simulink model "Problem3"  (R2020b)
settings: Solver=VariableStepAuto  StartTime=0.0  StopTime=0.1  RelTol=1e-3
settings Model: Creator=Saqlain  LastModifiedBy=Acer

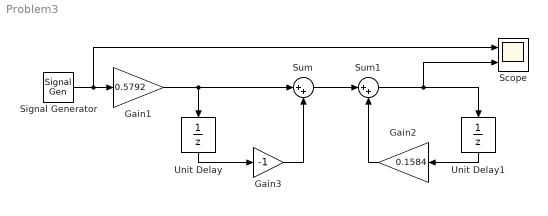
== system Problem3 ==
  Gain1 : Gain  Gain=0.5792
  Gain2 : Gain  Gain=0.1584
  Gain3 : Gain  Gain=-1
  Scope : Scope  NumInputPorts=2
  Signal Generator : SignalGenerator  Frequency=0.5
  Sum : Sum  Inputs=|++
  Sum1 : Sum  Inputs=|++
  Unit Delay : UnitDelay  SampleTime=-1  HasFrameUpgradeWarning=on
  Unit Delay1 : UnitDelay  SampleTime=-1  HasFrameUpgradeWarning=on
  wires:
  Sum/1 -> Sum1/1
  Gain3/1 -> Sum/2
  Unit Delay/1 -> Gain3/1
  Gain2/1 -> Sum1/2
  Unit Delay1/1 -> Gain2/1
  Signal Generator/1 -> Scope/1, Gain1/1
  Sum1/1 -> Unit Delay1/1, Scope/2
  Gain1/1 -> Sum/1, Unit Delay/1
